simulink model "Git_FSAE_FOC_SIM"  (R2025a)
settings: Solver=ode3  StartTime=0.0  StopTime=101.26  FixedStep=0.00933  RelTol=1e-3
libraries: slpidlib x2
settings Model: Creator=colin  LastModifiedBy=colin

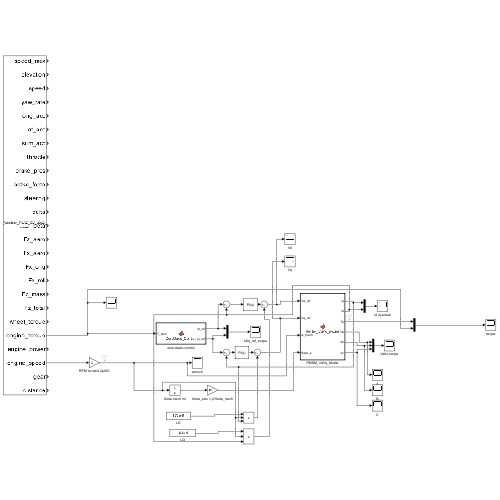
[thumbnail: Simulink's stored preview of the top-level diagram]
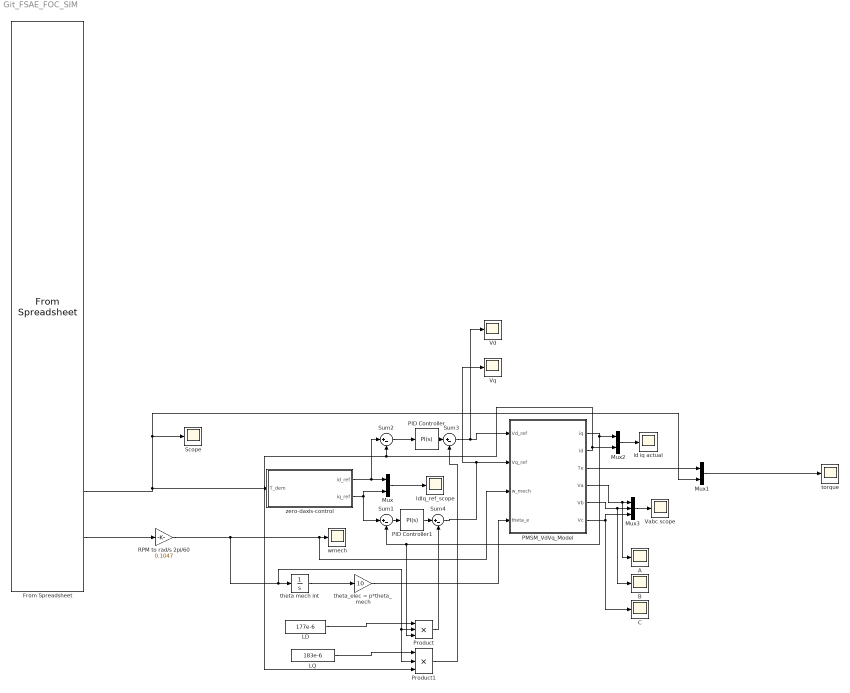
== system Git_FSAE_FOC_SIM ==
  A : Scope
      settings: ActiveDisplayYMinimum=45.201450941978493  ActiveDisplayYMaximum=248.76586485823418  DataLoggingVariableName=ScopeData6
  B : Scope
      settings: ActiveDisplayYMinimum=-56.537943910814576  ActiveDisplayYMaximum=-30.441126783042282  DataLoggingVariableName=ScopeData7
  C : Scope
      settings: DataLoggingVariableName=ScopeData8
  From Spreadsheet : FromSpreadsheet  FileName=Copy of OpenLAP_U_Windsor_FSAE_EV_2026_2019 Endurance.xlsx  SheetName=sheet
  IdIq_ref_scope : Scope
      settings: ActiveDisplayYMinimum=-1  ActiveDisplayYMaximum=1  DataLoggingVariableName=ScopeData3
  LD : Constant  Value=177e-6
  LQ : Constant  Value=183e-6
  Mux : Mux  Inputs=2
  Mux1 : Mux  Inputs=2
  Mux2 : Mux  Inputs=2
  Mux3 : Mux  Inputs=3
  PID Controller : slpidlib/PID Controller  Controller=PI  Form=Parallel  TimeDomain=Continuous-time  UseExternalTs=off  SampleTime=-1  IntegratorMethod=Forward Euler  FilterMethod=Forward Euler  ControllerParametersSource=internal  P=2*pi*500*177e-6  I=2*pi*500*0.0167  UseKiTs=off  D=0  UseExternalDerivativeSource=off  N=100  UseFilter=on  TunerSelectOption=Transfer Function Based (PID Tuner App)  InitialConditionSource=internal  InitialConditionForIntegrator=0  InitialConditionForFilter=0  DifferentiatorICPrevScaledInput=0  ExternalReset=none  TrackingMode=off  Kt=1  LimitOutput=off  SatLimitsSource=internal  UpperSaturationLimit=inf  LowerSaturationLimit=-inf  LinearizeAsGain=on  AntiWindupMode=none  Kb=1  LimitIntegrator=off  UpperIntegratorSaturationLimit=inf  LowerIntegratorSaturationLimit=-inf  POutMin=[]  POutMax=[]  IOutMin=[]  IOutMax=[]  DOutMin=[]  DOutMax=[]  NOutMin=[]  NOutMax=[]  SumOutMin=[]  SumOutMax=[]  SaturationOutMin=[]  SaturationOutMax=[]  PParamMin=[]  PParamMax=[]  IParamMin=[]  IParamMax=[]  DParamMin=[]  DParamMax=[]  NParamMin=[]  NParamMax=[]  KbParamMin=[]  KbParamMax=[]  KtParamMin=[]  KtParamMax=[]  KbOutMin=[]  KbOutMax=[]  KtOutMin=[]  KtOutMax=[]  IntegratorOutMin=[]  IntegratorOutMax=[]  FilterOutMin=[]  FilterOutMax=[]  SumI1OutMin=[]  SumI1OutMax=[]  SumI2OutMin=[]  SumI2OutMax=[]  SumI3OutMin=[]  SumI3OutMax=[]  SumI4OutMin=[]  SumI4OutMax=[]  SumDOutMin=[]  SumDOutMax=[]  DifferentiatorOutMin=[]  DifferentiatorOutMax=[]  FilterDiffOutCoefMin=[]  FilterDiffOutCoefMax=[]  ReciprocalOutMin=[]  ReciprocalOutMax=[]  SumDenOutMin=[]  SumDenOutMax=[]  SumNumOutMin=[]  SumNumOutMax=[]  DivideOutMin=[]  DivideOutMax=[]  UdiffTsProdOutMin=[]  UdiffTsProdOutMax=[]  NTsProdOutMin=[]  NTsProdOutMax=[]  UintegralTsProdOutMin=[]  UintegralTsProdOutMax=[]  UngainTsProdOutMin=[]  UngainTsProdOutMax=[]  ClampingZeroOutDataTypeStr=Inherit: Inherit via back propagation  ClampingZeroOutMin=[]  ClampingZeroOutMax=[]  FilterDenConstantOutDataTypeStr=Inherit: Inherit via back propagation  FilterDenConstantOutMin=[]  FilterDenConstantOutMax=[]  PCopyOutDataTypeStr=Inherit: Inherit via back propagation  PCopyOutMin=[]  PCopyOutMax=[]  NCopyOutDataTypeStr=Inherit: Inherit via back propagation  NCopyOutMin=[]  NCopyOutMax=[]  IntegratorContinuousStateAttributes=''  IntegratorStateMustResolveToSignalObject=off  IntegratorRTWStateStorageClass=Auto  FilterContinuousStateAttributes=''  FilterStateMustResolveToSignalObject=off  FilterRTWStateStorageClass=Auto  ParallelPVariant=InternalParameters  IdealPVariant=Disabled  IVariant=InternalParameters  DVariant=Disabled  IntegratorVariant=Continuous  SatVariant=Disabled  AWVariant=Passthrough  PCopyVariant=Disabled  TRVariant=Disabled  FdbkBlocksVariant=Forward  IdealPFdbkVariant=Disabled  SatFdbkVariant=Disabled  DerivativeFilterVariant=Disabled  NVariant=Disabled  NCopyVariant=Disabled_SignalSpec  FilterICVariant=Disabled  IntegratorICVariant=InternalICs  ExternalResetVariant=Disabled  TRSumVariant=Passthrough  SumFdbkVariant=Disabled  SumVariant=Sum_PI  TsampFilterVariant=InternalTs  TsampNgainVariant=Passthrough  TsampIntegralVariant=Disabled_SignalSpec  ExternalSaturationOutDataTypeStr=Inherit: Same as second input  DerivativeSourceVariant=Disabled  PreIntVariant=InternalPreInt
  PID Controller1 : slpidlib/PID Controller  Controller=PI  Form=Parallel  TimeDomain=Continuous-time  UseExternalTs=off  SampleTime=-1  IntegratorMethod=Forward Euler  FilterMethod=Forward Euler  ControllerParametersSource=internal  P=2*pi*500*177e-6  I=2*pi*500*0.0167  UseKiTs=off  D=0  UseExternalDerivativeSource=off  N=100  UseFilter=on  TunerSelectOption=Transfer Function Based (PID Tuner App)  InitialConditionSource=internal  InitialConditionForIntegrator=0  InitialConditionForFilter=0  DifferentiatorICPrevScaledInput=0  ExternalReset=none  TrackingMode=off  Kt=1  LimitOutput=off  SatLimitsSource=internal  UpperSaturationLimit=inf  LowerSaturationLimit=-inf  LinearizeAsGain=on  AntiWindupMode=none  Kb=1  LimitIntegrator=off  UpperIntegratorSaturationLimit=inf  LowerIntegratorSaturationLimit=-inf  POutMin=[]  POutMax=[]  IOutMin=[]  IOutMax=[]  DOutMin=[]  DOutMax=[]  NOutMin=[]  NOutMax=[]  SumOutMin=[]  SumOutMax=[]  SaturationOutMin=[]  SaturationOutMax=[]  PParamMin=[]  PParamMax=[]  IParamMin=[]  IParamMax=[]  DParamMin=[]  DParamMax=[]  NParamMin=[]  NParamMax=[]  KbParamMin=[]  KbParamMax=[]  KtParamMin=[]  KtParamMax=[]  KbOutMin=[]  KbOutMax=[]  KtOutMin=[]  KtOutMax=[]  IntegratorOutMin=[]  IntegratorOutMax=[]  FilterOutMin=[]  FilterOutMax=[]  SumI1OutMin=[]  SumI1OutMax=[]  SumI2OutMin=[]  SumI2OutMax=[]  SumI3OutMin=[]  SumI3OutMax=[]  SumI4OutMin=[]  SumI4OutMax=[]  SumDOutMin=[]  SumDOutMax=[]  DifferentiatorOutMin=[]  DifferentiatorOutMax=[]  FilterDiffOutCoefMin=[]  FilterDiffOutCoefMax=[]  ReciprocalOutMin=[]  ReciprocalOutMax=[]  SumDenOutMin=[]  SumDenOutMax=[]  SumNumOutMin=[]  SumNumOutMax=[]  DivideOutMin=[]  DivideOutMax=[]  UdiffTsProdOutMin=[]  UdiffTsProdOutMax=[]  NTsProdOutMin=[]  NTsProdOutMax=[]  UintegralTsProdOutMin=[]  UintegralTsProdOutMax=[]  UngainTsProdOutMin=[]  UngainTsProdOutMax=[]  ClampingZeroOutDataTypeStr=Inherit: Inherit via back propagation  ClampingZeroOutMin=[]  ClampingZeroOutMax=[]  FilterDenConstantOutDataTypeStr=Inherit: Inherit via back propagation  FilterDenConstantOutMin=[]  FilterDenConstantOutMax=[]  PCopyOutDataTypeStr=Inherit: Inherit via back propagation  PCopyOutMin=[]  PCopyOutMax=[]  NCopyOutDataTypeStr=Inherit: Inherit via back propagation  NCopyOutMin=[]  NCopyOutMax=[]  IntegratorContinuousStateAttributes=''  IntegratorStateMustResolveToSignalObject=off  IntegratorRTWStateStorageClass=Auto  FilterContinuousStateAttributes=''  FilterStateMustResolveToSignalObject=off  FilterRTWStateStorageClass=Auto  ParallelPVariant=InternalParameters  IdealPVariant=Disabled  IVariant=InternalParameters  DVariant=Disabled  IntegratorVariant=Continuous  SatVariant=Disabled  AWVariant=Passthrough  PCopyVariant=Disabled  TRVariant=Disabled  FdbkBlocksVariant=Forward  IdealPFdbkVariant=Disabled  SatFdbkVariant=Disabled  DerivativeFilterVariant=Disabled  NVariant=Disabled  NCopyVariant=Disabled_SignalSpec  FilterICVariant=Disabled  IntegratorICVariant=InternalICs  ExternalResetVariant=Disabled  TRSumVariant=Passthrough  SumFdbkVariant=Disabled  SumVariant=Sum_PI  TsampFilterVariant=InternalTs  TsampNgainVariant=Passthrough  TsampIntegralVariant=Disabled_SignalSpec  ExternalSaturationOutDataTypeStr=Inherit: Same as second input  DerivativeSourceVariant=Disabled  PreIntVariant=InternalPreInt
  PMSM_VdVq_Model : MATLAB Function  TreatAsAtomicUnit=on
  Product : Product  Inputs=3
  Product1 : Product  Inputs=3
  RPM to rad/s 2pi/60 : Gain  Gain=0.1047
  Scope : Scope
      settings: ActiveDisplayYMinimum=-22.263945308586713  ActiveDisplayYMaximum=200.37550777728046  DataLoggingVariableName=ScopeData4
  Sum{1..4} (4 alike) : Sum  Inputs=|+-
  Vabc scope : Scope
      settings: ActiveDisplayYMinimum=-382.04324328865988  ActiveDisplayYMaximum=400.9834820684564  DataLoggingVariableName=ScopeData2
  Vd : Scope
      settings: ActiveDisplayYMinimum=-1  ActiveDisplayYMaximum=1  DataLoggingVariableName=ScopeData9
  Vq : Scope
      settings: ActiveDisplayYMinimum=-1  ActiveDisplayYMaximum=1  DataLoggingVariableName=ScopeData10
  id iq actual : Scope
      settings: ActiveDisplayYMinimum=-41.833181080408437  ActiveDisplayYMaximum=317.51937925293242
  theta mech int : Integrator
  theta_elec = p*theta_mech : Gain  Gain=10
  torque : Scope
      settings: ActiveDisplayYMinimum=-209.33831772546404  ActiveDisplayYMaximum=221.89997260148306  DataLoggingVariableName=ScopeData11
  wmech : Scope
      settings: ActiveDisplayYMinimum=-1  ActiveDisplayYMaximum=1  DataLoggingVariableName=ScopeData5
  zero-daxis-control : MATLAB Function  TreatAsAtomicUnit=on
  wires:
  zero-daxis-control/1(id_ref) -> Sum2/1, Mux/1
  theta mech int/1 -> theta_elec = p*theta_mech/1
  Mux/1 -> IdIq_ref_scope/1
  zero-daxis-control/2(iq_ref) -> Sum1/1, Mux/2
  Sum1/1 -> PID Controller1/1
  Sum2/1 -> PID Controller/1
  theta_elec = p*theta_mech/1 -> PMSM_VdVq_Model/4(theta_e)
  PMSM_VdVq_Model/1(iq) -> Mux2/1, Product/3, Sum1/2
  PMSM_VdVq_Model/2(id) -> Mux2/2, Product1/3, Sum2/2
  PMSM_VdVq_Model/3(Te) -> Mux1/1
  Mux1/1 -> torque/1
  Mux2/1 -> id iq actual/1
  PMSM_VdVq_Model/4(Va) -> A/1, Mux3/1
  PMSM_VdVq_Model/5(Vb) -> Mux3/2, B/1
  PMSM_VdVq_Model/6(Vc) -> C/1, Mux3/3
  Mux3/1 -> Vabc scope/1
  Sum3/1 -> Vd/1, PMSM_VdVq_Model/1(Vd_ref)
  Sum4/1 -> Vq/1, PMSM_VdVq_Model/2(Vq_ref)
  PID Controller1/1 -> Sum4/1
  PID Controller/1 -> Sum3/1
  Product/1 -> Sum4/2
  Product1/1 -> Sum3/2
  LD/1 -> Product/1
  LQ/1 -> Product1/1
  From Spreadsheet/21 -> Mux1/2, Scope/1, zero-daxis-control/1(T_dem)
  From Spreadsheet/23 -> RPM to rad/s 2pi/60/1
  RPM to rad/s 2pi/60/1 -> Product1/2, Product/2, theta mech int/1, PMSM_VdVq_Model/3(w_mech), wmech/1

== matlab function Git_FSAE_FOC_SIM/zero-daxis-control ==
  data: T_dem input; id_ref output; iq_ref output
function [id_ref, iq_ref] = ZeroDaxis_Control(T_dem)

Kt = 0.94;

% ---- SET PER EVENT ----
Iq_max_RMS  = 235;   % Acceleration / Autocross
% Iq_max_RMS = 120;  % Endurance / Skidpad

Iq_min_RMS = -120;

iq_dem_RMS = T_dem / Kt;

if iq_dem_RMS > Iq_max_RMS
    iq_dem_RMS = Iq_max_RMS;
elseif iq_dem_RMS < Iq_min_RMS
    iq_dem_RMS = Iq_min_RMS;
end

iq_ref = iq_dem_RMS;
id_ref = 0;
end

== matlab function Git_FSAE_FOC_SIM/PMSM_VdVq_Model ==
  data: Vd_ref input; iq output; Vq_ref input; w_mech input; theta_e input; id output; Te output; Va output; Vb output; Vc output
function [iq, id, Te, Va, Vb, Vc] = PMSM_VdVq_Model(Vd_ref, Vq_ref, w_mech, theta_e)
% Steady-state dq PMSM model + inverse Park/Clarke
% Inputs:
%  Vd_ref, Vq_ref : d-q voltages [V]
%  w_mech         : mechanical speed [rad/s]
%  theta_e        : electrical angle [rad]
%
% Outputs:
%  iq, id         : d-q currents [A_peak]
%  Te             : electromagnetic torque [Nm]
%  Va, Vb, Vc     : phase voltages [V]
% Motor parameters (rough starting values, tune later from datasheet)
p    = 10;           % pole pairs
Rs   = 0.0167;       % stator phase resistance [Ohm]
Ld   = 177e-6;      % d-axis inductance [H]
Lq   = 183e-6;      % q-axis inductance [H]
Kt   = 0.94;        % torque constant [Nm/A_RMS]
psi_f = Kt / p;  % flux linkage [Wb]

% Electrical speed
w_e = p * w_mech;   % [rad/s]

% Avoid division issues at zero speed
if abs(w_e) < 1e-3
    w_e = sign(w_e) * 1e-3;
end

% Solve steady-state dq equations
% [ Rs      -w_e*Lq ] [id] = [ Vd_ref           ]
% [ w_e*Ld   Rs     ] [iq]   [ Vq_ref - w_e*psi_f]
A = [Rs,       -w_e*Lq;
     w_e*Ld,    Rs     ];
b = [Vd_ref;
     Vq_ref - w_e*psi_f];

x = A \ b;
id = x(1);
iq = x(2);

% Electromagnetic torque
Te = p * (psi_f*iq + (Ld - Lq)*id*iq);

% --- Inverse Park: dq -> alpha-beta (using voltages) ---
c = cos(theta_e);
s = sin(theta_e);

Valpha =  Vd_ref*c - Vq_ref*s;
Vbeta  =  Vd_ref*s + Vq_ref*c;

% --- Inverse Clarke: alpha-beta -> a-b-c ---
Va = Valpha;
Vb = -0.5*Valpha + sqrt(3)/2 * Vbeta;
Vc = -0.5*Valpha - sqrt(3)/2 * Vbeta;
end
